simulink model "setepb_d"  (R2024a)
settings: Solver=VariableStepAuto  StartTime=0.0  StopTime=10.0  RelTol=1e-3
settings Model: Creator=mustafaenesozdel  LastModifiedBy=mustafaenesozdel

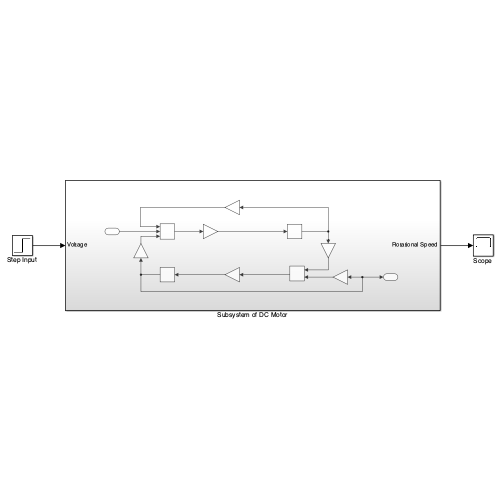
[thumbnail: Simulink's stored preview of the top-level diagram]
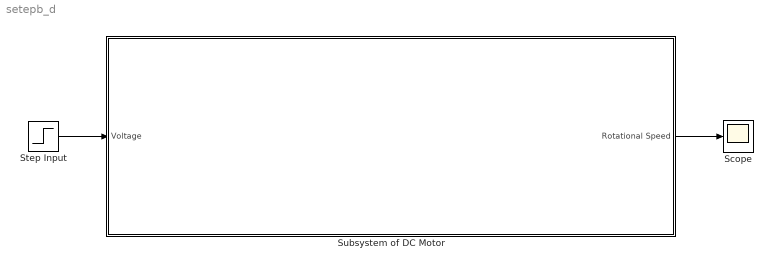
== system setepb_d ==
  Scope : Scope
  Step Input : Step  Time=0.0001  SampleTime=0
  Subsystem of DC Motor : Subsystem
  wires:
  Step Input/1 -> Subsystem of DC Motor/1(Voltage)
  Subsystem of DC Motor/1(Rotational Speed) -> Scope/1

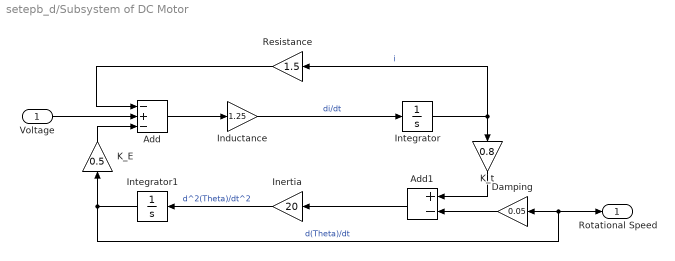
== system setepb_d/Subsystem of DC Motor ==
  Voltage : Inport
  Add : Sum  Inputs=-+-
  Add1 : Sum  Inputs=+-
  Damping : Gain  Gain=0.05
  Inductance : Gain  Gain=1.25
  Inertia : Gain  Gain=20
  Integrator : Integrator
  Integrator1 : Integrator
  K_E : Gain  Gain=0.5
  K_t : Gain  Gain=0.8
  Resistance : Gain  Gain=1.5
  Rotational Speed : Outport
  wires:
  Voltage/1 -> Add/2
  Damping/1 -> Add1/2
  K_t/1 -> Add1/1
  Inductance/1 -> Integrator/1  "di/dt"
  Integrator/1 -> Resistance/1, K_t/1  "i"
  K_E/1 -> Add/3
  Inertia/1 -> Integrator1/1  "d^2(Theta)/dt^2"
  Add/1 -> Inductance/1
  Resistance/1 -> Add/1
  Integrator1/1 -> Rotational Speed/1, Damping/1, K_E/1  "d(Theta)/dt"
  Add1/1 -> Inertia/1
